simulink model "DRI_furnace"  (R2023b)
settings: Solver=ode15s  StartTime=0.0  StopTime=3600*24
values from neighbouring files (symbols this model uses):
  a_b = 6*(1-eps_bed)/(r_p*2)    (= 200)    [DRI_furnace_loader.m]
  A_furnace = pi*r_furnace^2    (= 23.7582944428)    [DRI_furnace_loader.m]
  A_furnace_pel = A_furnace*(1-eps_bed)    (= 11.8791472214)    [DRI_furnace_loader.m]
  A_wall = (2*pi*r_furnace*dz)    [DRI_furnace_loader.m]
  c_CH4init = interp1([1:1:length(c_CH4init)],c_CH4init, linspace(1,length(c_CH4init),n_furnace))    [DRI_furnace_loader.m]    (also in inital_conditions.m = out.CH4_conc.data(end,:); initcond.mat = [1.85705986545 1.89555733619 1.89749367615 1.89250716351 1.8; initcond_H2.mat = [-5.10200321778e-23 -5.14631233267e-23 -5.19105613109e-23 -5; initcond_NG.mat = [1.53547326032 1.50495486962 1.48970115024 1.4755028102 1.46)
  c_Cinit = interp1([1:1:length(c_Cinit)],c_Cinit, linspace(1,length(c_Cinit),n_furnace))    [DRI_furnace_loader.m]    (also in inital_conditions.m = out.C_conc.data(end,:); initcond.mat = [3.21457388191e-26 -1.33944556404e-26 -9.41053781484e-33 -9.; initcond_H2.mat = [-3.07981965757e-283 -7.05821276017e-284 -1.12151880238e-284; initcond_NG.mat = [40.5707549093 38.5039319297 36.8451113121 35.2570306703 33.)
  c_CO2init = interp1([1:1:length(c_CO2init)],c_CO2init, linspace(1,length(c_CO2init),n_furnace))    [DRI_furnace_loader.m]    (also in inital_conditions.m = out.CO2_conc.data(end,:); initcond.mat = [0.424855142623 0.487573768012 0.610878568601 0.778581871411; initcond_H2.mat = [8.08256932825e-22 8.11925418298e-22 8.15917924386e-22 8.201; initcond_NG.mat = [0.33936960913 0.362161667495 0.389241162314 0.417886502664 )
  c_COinit = interp1([1:1:length(c_COinit)],c_COinit, linspace(1,length(c_COinit),n_furnace))    [DRI_furnace_loader.m]    (also in inital_conditions.m = out.CO_conc.data(end,:); initcond.mat = [5.62429774676 5.68698007947 5.56998267729 5.3860363993 5.16; initcond_H2.mat = [-3.5707332813e-22 -3.59888147715e-22 -3.62743836785e-22 -3.; initcond_NG.mat = [7.01547259829 7.0384402498 7.00998897858 6.97797046171 6.94)
  c_Fe2O3init = interp1([1:1:length(c_Fe2O3init)],c_Fe2O3init, linspace(1,length(c_Fe2O3init),n_furnace))    [DRI_furnace_loader.m]    (also in inital_conditions.m = out.Fe2O3_conc.data(end,:); initcond.mat = [845.154140842 845.181508816 845.220501809 845.323312901 845; initcond_H2.mat = [-0.0380770099519 -0.0370367139242 -0.0360185883395 -0.03502; initcond_NG.mat = [-0.0405281021674 -0.0396025120519 -0.0386898228266 -0.03778)
  c_Fe3O4init = interp1([1:1:length(c_Fe3O4init)],c_Fe3O4init, linspace(1,length(c_Fe3O4init),n_furnace))    [DRI_furnace_loader.m]    (also in inital_conditions.m = out.Fe3O4_conc.data(end,:); initcond.mat = [826.123395955 826.094631755 826.211564736 834.377927258 899; initcond_H2.mat = [0.0321426182211 0.0314818734285 0.030826675132 0.0301767421; initcond_NG.mat = [0.0360465051239 0.0353534026747 0.0346647730928 0.033980211)
  c_Feinit = interp1([1:1:length(c_Feinit)],c_Feinit, linspace(1,length(c_Feinit),n_furnace))    [DRI_furnace_loader.m]    (also in inital_conditions.m = out.Fe_conc.data(end,:); initcond.mat = [836.997845525 830.524010614 758.675200979 644.11637995 545.; initcond_H2.mat = [2198.89990701 2151.53921086 2100.32127816 2045.76128409 198; initcond_NG.mat = [2217.04023267 2190.22219582 2162.02573698 2132.25158626 210)
  c_FeOinit = interp1([1:1:length(c_FeOinit)],c_FeOinit, linspace(1,length(c_FeOinit),n_furnace))    [DRI_furnace_loader.m]    (also in inital_conditions.m = out.FeO_conc.data(end,:); initcond.mat = [523.921847425 532.250412357 624.547839148 764.836368397 835; initcond_H2.mat = [239.269098944 300.197811145 366.088832018 436.279393422 510; initcond_NG.mat = [215.930334993 250.431267245 286.705532207 325.009485154 365)
  c_H2init = interp1([1:1:length(c_H2init)],c_H2init, linspace(1,length(c_H2init),n_furnace))    [DRI_furnace_loader.m]    (also in inital_conditions.m = out.H2_conc.data(end,:); initcond.mat = [8.579601171 8.64686368664 8.51185743267 8.39999947053 8.265; initcond_H2.mat = [17.2543528358 17.2782610911 17.296864644 17.3099892036 17.3; initcond_NG.mat = [11.1435961113 11.2383917061 11.232749456 11.2204098296 11.2)
  c_H2Oinit = interp1([1:1:length(c_H2Oinit)],c_H2Oinit, linspace(1,length(c_H2Oinit),n_furnace))    [DRI_furnace_loader.m]    (also in inital_conditions.m = out.H2O_conc.data(end,:); initcond.mat = [0.757633216435 0.883934685646 1.02867679163 1.11546273638 1; initcond_H2.mat = [0.442325343528 0.548013106661 0.662035872616 0.783558475201; initcond_NG.mat = [0.493575761349 0.511052154474 0.544598386657 0.580268512829)
  c_N2init = interp1([1:1:length(c_N2init)],c_N2init, linspace(1,length(c_N2init),n_furnace))    [DRI_furnace_loader.m]    (also in inital_conditions.m = out.N2_conc.data(end,:); initcond.mat = [0.304985476887 0.311307927602 0.311625933271 0.310806996864; initcond_H2.mat = [0.335892697728 0.338352501527 0.340869822099 0.343425499389; initcond_NG.mat = [0.34370092648 0.344898196415 0.344837358554 0.344718971495 )
  DRIflow = 45.1    [DRI_furnace_loader.m]
  dz = flip(diff(dzfun))    [DRI_furnace_loader.m]
  eps_bed = 0.5    [DRI_furnace_loader.m]
  MM_C = 12.011/1000    (= 0.012011)    [DRI_furnace_loader.m]
  MM_CH4 = 16.04    [DRI_furnace_loader.m]
  MM_CO = 28.01    [DRI_furnace_loader.m]
  MM_CO2 = 44.01    [DRI_furnace_loader.m]
  MM_Fe = 55.845/1000    (= 0.055845)    [DRI_furnace_loader.m]    (also in iron_props.m)
  MM_Fe2O3 = 159.69/1000    (= 0.15969)    [DRI_furnace_loader.m]    (also in iron_props.m)
  MM_Fe3O4 = 251.53/1000    (= 0.25153)    [DRI_furnace_loader.m]    (also in iron_props.m)
  MM_FeO = 71.844/1000    (= 0.071844)    [DRI_furnace_loader.m]    (also in iron_props.m)
  MM_Gan = 60.08/1000    (= 0.06008)    [DRI_furnace_loader.m]
  MM_H2 = 2.016    [DRI_furnace_loader.m]
  MM_H2O = 18.015    [DRI_furnace_loader.m]
  MM_N2 = 28.013    [DRI_furnace_loader.m]
  mol_Fe2O3init = rho_p*0.9665/MM_Fe2O3*V_s(2:end)    [DRI_furnace_loader.m]    (also in inital_conditions.m = out.mol_Fe2O3init.data(end,:); initcond.mat = [61783.2992712 61783.2992712 61783.2992712 61783.2992712 617)
  n_furnace = 25    [DRI_furnace_loader.m]
  ndotinit = interp1([1:1:length(ndotinit)],ndotinit, linspace(1,length(ndotinit),n_furnace))    [DRI_furnace_loader.m]    (also in inital_conditions.m = out.ndot.data(end,:); initcond.mat = [2210.71780913 2256.54672706 2258.85182304 2252.91568039 224; initcond_H2.mat = [2085.86199266 2093.15115329 2100.66626347 2108.33970255 211; initcond_NG.mat = [2330.74775425 2364.28126123 2378.87094646 2385.81987377 238)
  nr1init = ones(size(T_ginit))*33375    [DRI_furnace_loader.m]    (also in inital_conditions.m = out.nr1.data(end,:); initcond.mat = [61803.8716376 61802.685448 61800.9961847 61796.5422507 6178; initcond_H2.mat = [17138.8276975 17138.822469 17138.817352 17138.8123408 17138; initcond_NG.mat = [34277.6800528 34277.6707483 34277.6615734 34277.652487 3427)
  nr2init = ones(size(T_ginit))*22119    [DRI_furnace_loader.m]    (also in inital_conditions.m = out.nr2.data(end,:); initcond.mat = [41188.8753355 41188.8526513 41178.4232644 40740.5447947 379; initcond_H2.mat = [11425.7737029 11425.772508 11425.7713681 11425.7702806 1142; initcond_NG.mat = [22851.536777 22851.5353796 22851.5340375 22851.5327263 2285)
  nr3init = ones(size(T_ginit))*63083    [DRI_furnace_loader.m]    (also in inital_conditions.m = out.nr3.data(end,:); initcond.mat = [123566.152328 121180.275703 99887.5755955 72587.2577367 536; initcond_H2.mat = [31604.1937028 30923.4912249 30187.3497294 29403.1736897 285; initcond_NG.mat = [63729.8393954 62958.9426131 62148.4224578 61292.5508252 603)
  R = 8.314    [Bou.m]    (also in DRI_furnace_loader.m; G_CO.m; MD.m; SMR.m)
  r_furnace = 2.75    [DRI_furnace_loader.m]
  r_p = 15e-3/2    (= 0.0075)    [DRI_furnace_loader.m]
  Reducerflow = 2228.1*(x_H2in*MM_H2 + x_COin*MM_CO + x_H2Oin*MM_H2O +x_CO2in*MM_CO2 + x_N2in*MM_N2 + x_CH4in*MM_CH4)/1000    (= 31.1426394672)    [DRI_furnace_loader.m]
  rho_p = 3528    [DRI_furnace_loader.m]
  T_ginit = interp1([1:1:length(T_ginit)],T_ginit, linspace(1,length(T_ginit),n_furnace))    [DRI_furnace_loader.m]    (also in inital_conditions.m = out.T_g.data(end,:); initcond.mat = [1196.67659973 1106.80014704 1071.61124107 1050.32194229 103; initcond_H2.mat = [1206.04002008 1196.92003246 1187.72467669 1178.52571193 116; initcond_NG.mat = [1059.94701026 1050.97990802 1047.95611626 1045.20600654 104)
  T_sinit = interp1([1:1:length(T_sinit)],T_sinit, linspace(1,length(T_sinit),n_furnace))    [DRI_furnace_loader.m]    (also in inital_conditions.m = out.T_s.data(end,:); initcond.mat = [1154.91557113 1100.93660653 1069.19977285 1049.37027984 104; initcond_H2.mat = [1198.21532505 1188.90892541 1179.58573027 1170.31082456 116; initcond_NG.mat = [1055.14966191 1048.70059171 1045.82868823 1043.13322913 104)
  V_g = (4/3)*pi*r_p^3*n_pellets_dz*(eps_bed/(1-eps_bed))    [DRI_furnace_loader.m]
  V_p = 4/3*pi*r_p^3    (= 1.76714586764e-06)    [DRI_furnace_loader.m]
  V_s = (4/3)*pi*r_p^3*n_pellets_dz    [DRI_furnace_loader.m]
  x_CH4in = 0.105824828    [DRI_furnace_loader.m]
  x_CO2in = 0.024    [DRI_furnace_loader.m]
  x_COin = 0.320711862    [DRI_furnace_loader.m]
  x_H2in = 0.489526511    [DRI_furnace_loader.m]
  x_H2Oin = 0.042557156    [DRI_furnace_loader.m]
  x_N2in = 0.017379642    [DRI_furnace_loader.m]
libraries: simulink x1
(part 1 of 2)
settings Model: Creator=jimmonen  LastModifiedBy=jimmonen
settings SolverCC: AlgebraicLoopSolver=TrustRegion
settings DebuggingCC: UnconnectedInputMsg=warning  UnconnectedOutputMsg=warning  UnconnectedLineMsg=warning
settings ModelReferenceCC: EnableRefExpFcnMdlSchedulingChecks=on
settings RTWCC: DLArmComputeVersion=19.05

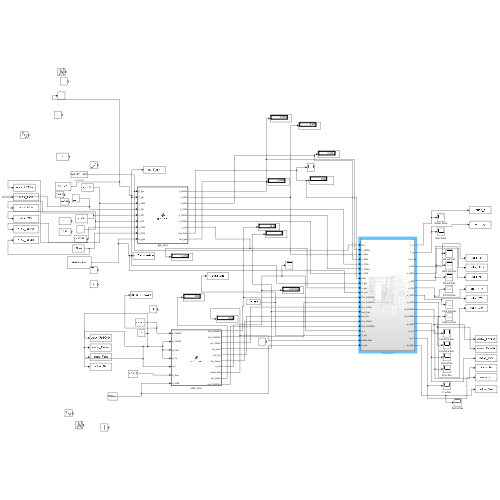
[thumbnail: Simulink's stored preview of the top-level diagram]
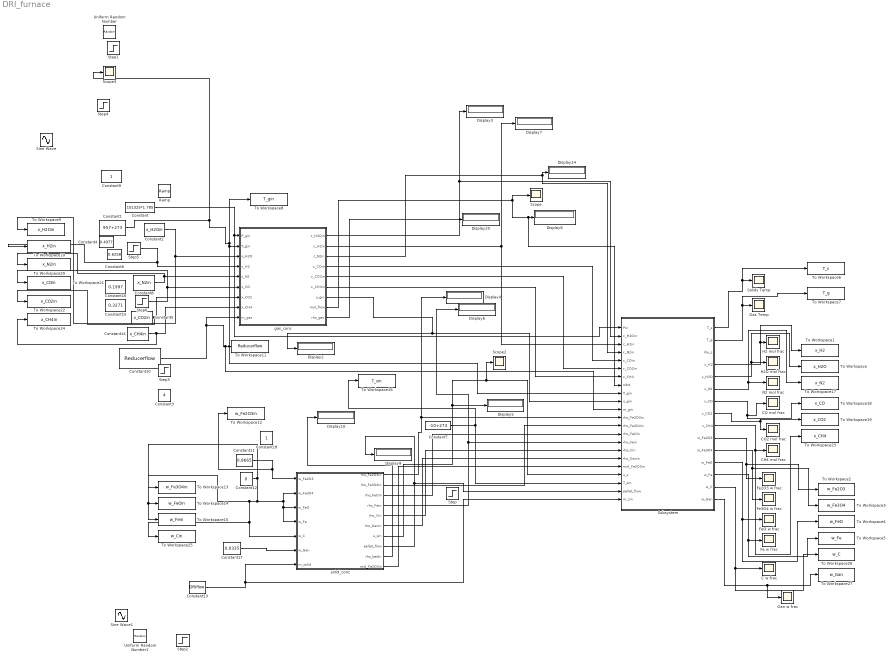
== system DRI_furnace ==
  C w frac : Scope
  CH4 mol frac : Scope
  CO mol frac : Scope
  CO2 mol frac : Scope
  Constant : Constant  Value=101325*1.785
  Constant1 : Constant  Value=957+273
  Constant10 : Constant  Value=Reducerflow
  Constant11 : Constant  Value=0.9665
  Constant12 : Constant  Value=0
  Constant13 : Constant  Value=DRIflow
  Constant14 : Constant  Value=x_CH4in
  Constant15 : Constant  Value=0.3271
  Constant16 : Constant  Value=0.1997
  Constant17 : Constant  Value=0.0335
  Constant18 : Constant
  Constant2 : Constant  Value=x_H2Oin
  Constant3 : Constant  Value=4
  Constant4 : Constant  Value=0.4977
  Constant5 : Constant  Value=x_CO2in
  Constant6 : Constant  Value=0.6258
  Constant7 : Constant  Value=-10+273
  Constant8 : Constant  Value=x_N2in
  Constant9 : Constant
  Display{2..10,14,20} (11 alike) : Display
  Fe w frac : Scope
  Fe2O3 w frac : Scope
  Fe3O4 w frac : Scope
  FeO w frac : Scope
  Gan w frac : Scope
  Gas Temp : Scope
  H2 mol frac : Scope
  H2O mol frac : Scope
  N2 mol frac : Scope
  Ramp : simulink/Sources/Ramp  slope=-5/(3600)  start=3600  InitialOutput=800+273
  Scope : Scope
  Scope2 : Scope
  Scope3 : Scope
  Sine Wave : Sin  Amplitude=2  Bias=Reducerflow  Frequency=1/(3600*0.5)  SampleTime=0
  Sine Wave1 : Sin  Amplitude=15  Bias=52  Frequency=1/(3600*0.5)  SampleTime=0
  Solids Temp : Scope
  Step : Step  Time=3600*6  Before=4750  After=5000  SampleTime=0
  Step1 : Step  Time=3600*1  Before=800+273  After=700+273  SampleTime=0
  Step2 : Step  Time=3600*1  Before=DRIflow  After=DRIflow+25  SampleTime=0
  Step3 : Step  Time=3600*1  Before=Reducerflow  After=14.2236  SampleTime=0
  Step4 : Step  Time=3600*1  Before=0.98  After=0.9  SampleTime=0
  Step5 : Step  Time=3600*1  Before=x_H2in  After=x_H2in  SampleTime=0
  Step6 : Step  Time=3600*1  Before=x_COin  After=x_COin  SampleTime=0
  Subsystem : Subsystem
  To Workspace : ToWorkspace  VariableName=x_H2O  SaveFormat=Timeseries  SampleTime=-1
  To Workspace1 : ToWorkspace  VariableName=x_H2  SaveFormat=Timeseries  SampleTime=-1
  To Workspace10 : ToWorkspace  VariableName=x_H2in  SaveFormat=Timeseries  SampleTime=-1
  To Workspace11 : ToWorkspace  VariableName=Reducerflow  SaveFormat=Timeseries  SampleTime=-1
  To Workspace12 : ToWorkspace  VariableName=w_Fe2O3in  SaveFormat=Timeseries  SampleTime=-1
  To Workspace13 : ToWorkspace  VariableName=w_Fe3O4in  SaveFormat=Timeseries  SampleTime=-1
  To Workspace14 : ToWorkspace  VariableName=w_FeOin  SaveFormat=Timeseries  SampleTime=-1
  To Workspace15 : ToWorkspace  VariableName=w_Fein  SaveFormat=Timeseries  SampleTime=-1
  To Workspace16 : ToWorkspace  VariableName=T_sin  SaveFormat=Timeseries  SampleTime=-1
  To Workspace17 : ToWorkspace  VariableName=x_N2  SaveFormat=Timeseries  SampleTime=-1
  To Workspace18 : ToWorkspace  VariableName=x_CO  SaveFormat=Timeseries  SampleTime=-1
  To Workspace19 : ToWorkspace  VariableName=x_CO2  SaveFormat=Timeseries  SampleTime=-1
  To Workspace2 : ToWorkspace  VariableName=w_Fe2O3  SaveFormat=Timeseries  SampleTime=-1
  To Workspace20 : ToWorkspace  VariableName=x_N2in  SaveFormat=Timeseries  SampleTime=-1
  To Workspace21 : ToWorkspace  VariableName=x_COin  SaveFormat=Timeseries  SampleTime=-1
  To Workspace22 : ToWorkspace  VariableName=x_CO2in  SaveFormat=Timeseries  SampleTime=-1
  To Workspace23 : ToWorkspace  VariableName=x_CH4  SaveFormat=Timeseries  SampleTime=-1
  To Workspace24 : ToWorkspace  VariableName=x_CH4in  SaveFormat=Timeseries  SampleTime=-1
  To Workspace25 : ToWorkspace  VariableName=w_Cin  SaveFormat=Timeseries  SampleTime=-1
  To Workspace26 : ToWorkspace  VariableName=w_C  SaveFormat=Timeseries  SampleTime=-1
  To Workspace27 : ToWorkspace  VariableName=w_Gan  SaveFormat=Timeseries  SampleTime=-1
  To Workspace3 : ToWorkspace  VariableName=w_Fe3O4  SaveFormat=Timeseries  SampleTime=-1
  To Workspace4 : ToWorkspace  VariableName=w_FeO  SaveFormat=Timeseries  SampleTime=-1
  To Workspace5 : ToWorkspace  VariableName=w_Fe  SaveFormat=Timeseries  SampleTime=-1
  To Workspace6 : ToWorkspace  VariableName=T_s  SaveFormat=Timeseries  SampleTime=-1
  To Workspace7 : ToWorkspace  VariableName=T_g  SaveFormat=Timeseries  SampleTime=-1
  To Workspace8 : ToWorkspace  VariableName=T_gin  SaveFormat=Timeseries  SampleTime=-1
  To Workspace9 : ToWorkspace  VariableName=x_H2Oin  SaveFormat=Timeseries  SampleTime=-1
  Uniform Random Number : UniformRandomNumber  Minimum=800  Maximum=1000  SampleTime=3600
  Uniform Random Number1 : UniformRandomNumber  Minimum=DRIflow -7  Maximum=DRIflow +7  SampleTime=3600
  gas_conc : MATLAB Function  TreatAsAtomicUnit=on
  solid_conc : MATLAB Function  TreatAsAtomicUnit=on
  wires:
  gas_conc/1(c_H2Oin) -> Display3/1, Subsystem/2(c_H2Oin)
  gas_conc/2(c_H2in) -> Display7/1, Subsystem/3(c_H2in)
  gas_conc/3(c_N2in) -> Display14/1, Subsystem/4(c_N2in)
  solid_conc/1(rho_Fe2O3in) -> Display4/1, Subsystem/12(rho_Fe2O3in)
  Constant1/1 -> Subsystem/9(T_gin), gas_conc/2(T_gin), To Workspace8/1, Scope3/1
  Constant/1 -> Subsystem/1(Pin), gas_conc/1(P_gin)
  Constant10/1 -> gas_conc/9(m_gas), To Workspace11/1, Subsystem/11(m_gin)
  gas_conc/7(u_gin) -> Subsystem/10(u_gin), Display2/1
  Constant11/1 -> solid_conc/1(w_Fe2O3), To Workspace12/1
  solid_conc/4(rho_Fein) -> Display6/1, Subsystem/15(rho_Fein)
  solid_conc/7(u_sin) -> Scope2/1, Subsystem/19(u_s), Display5/1
  solid_conc/8(pellet_flow) -> Display9/1, Subsystem/21(pellet_flow)
  gas_conc/8(mol_flow) -> Display8/1, Subsystem/8(ndot), Scope/1
  solid_conc/9(rho_bedin) -> Display10/1
  gas_conc/9(rho_gas) -> Display20/1
  Subsystem/2(T_g) -> To Workspace7/1, Gas Temp/1
  Subsystem/1(T_s) -> To Workspace6/1, Solids Temp/1
  Constant7/1 -> To Workspace16/1, Subsystem/20(T_sin)
  solid_conc/2(rho_Fe3O4in) -> Subsystem/13(rho_Fe3O4in)
  solid_conc/3(rho_FeOin) -> Subsystem/14(rho_FeOin)
  Constant13/1 -> solid_conc/7(m_solid), Subsystem/22(m_sin)
  gas_conc/4(c_COin) -> Subsystem/5(c_COin)
  gas_conc/5(c_CO2in) -> Subsystem/6(c_CO2in)
  Step6/1 -> To Workspace21/1, gas_conc/6(x_CO)
  Constant5/1 -> gas_conc/7(x_CO2), To Workspace22/1
  Constant8/1 -> To Workspace20/1, gas_conc/5(x_N2)
  Step5/1 -> To Workspace10/1, gas_conc/4(x_H2)
  Constant2/1 -> To Workspace9/1, gas_conc/3(x_H2O)
  Subsystem/4(x_H2) -> To Workspace1/1, H2 mol frac/1
  Subsystem/5(x_H2O) -> To Workspace/1, H2O mol frac/1
  Subsystem/6(x_N2) -> To Workspace17/1, N2 mol frac/1
  Subsystem/7(x_CO) -> To Workspace18/1, CO mol frac/1
  Subsystem/8(x_CO2) -> CO2 mol frac/1, To Workspace19/1
  Subsystem/10(w_Fe2O3) -> Fe2O3 w frac/1, To Workspace2/1
  Subsystem/11(w_Fe3O4) -> Fe3O4 w frac/1, To Workspace3/1
  Subsystem/13(w_Fe) -> To Workspace5/1, Fe w frac/1
  Subsystem/12(w_FeO) -> To Workspace4/1, FeO w frac/1
  Subsystem/9(x_CH4) -> To Workspace23/1, CH4 mol frac/1
  Constant14/1 -> To Workspace24/1, gas_conc/8(x_CH4)
  gas_conc/6(c_CH4in) -> Subsystem/7(c_CH4)
  solid_conc/5(rho_Cin) -> Subsystem/16(rho_Cin)
  solid_conc/6(rho_Ganin) -> Subsystem/17(rho_Ganin)
  Constant12/1 -> solid_conc/5(w_C), To Workspace25/1, To Workspace15/1, To Workspace14/1, solid_conc/4(w_Fe), solid_conc/3(w_FeO), solid_conc/2(w_Fe3O4), To Workspace13/1
  Subsystem/14(w_C) -> To Workspace26/1, C w frac/1
  Constant17/1 -> solid_conc/6(w_Gan)
  Subsystem/15(w_Gan) -> Gan w frac/1, To Workspace27/1
  solid_conc/10(mol_Fe2O3in) -> Subsystem/18(mol_Fe2O3in)

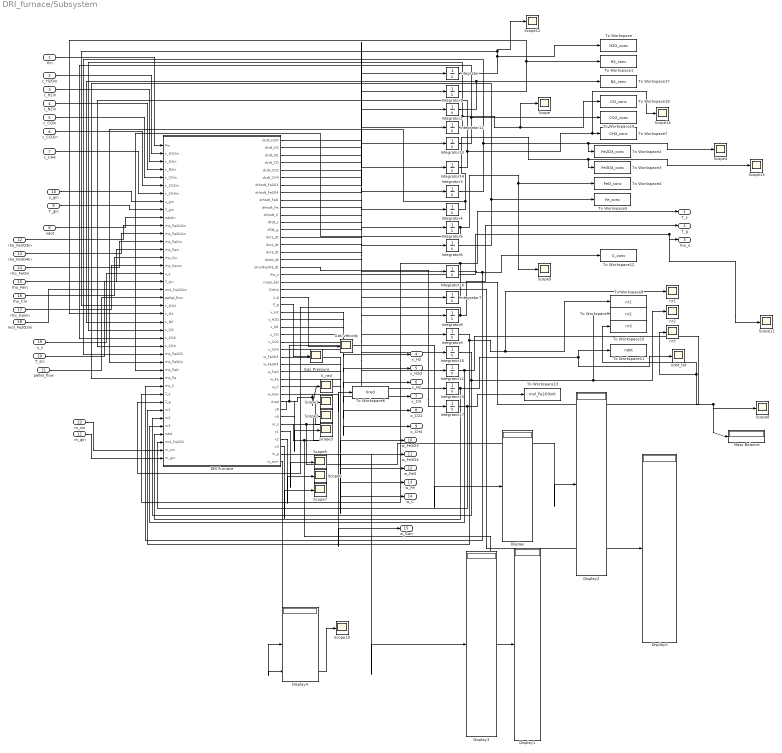
== system DRI_furnace/Subsystem ==
  Pin : Inport
  c_H2Oin : Inport  Port=2
  c_H2in : Inport  Port=3
  c_N2in : Inport  Port=4
  c_COin : Inport  Port=5
  c_CO2in : Inport  Port=6
  c_CH4 : Inport  Port=7
  ndot : Inport  Port=8
  T_gin : Inport  Port=9
  u_gin : Inport  Port=10
  m_gin : Inport  Port=11
  rho_Fe2O3in : Inport  Port=12
  rho_Fe3O4in : Inport  Port=13
  rho_FeOin : Inport  Port=14
  rho_Fein : Inport  Port=15
  rho_Cin : Inport  Port=16
  rho_Ganin : Inport  Port=17
  mol_Fe2O3in : Inport  Port=18
  u_s : Inport  Port=19
  T_sin : Inport  Port=20
  pellet_flow : Inport  Port=21
  m_sin : Inport  Port=22
  DRI Furnace : MATLAB Function  TreatAsAtomicUnit=on
  Display{,1..5} (6 alike) : Display
  Gas Pressure : Scope
  Gas Velocity : Scope
  Integrator : Integrator  InitialCondition=c_H2Oinit
  Integrator1 : Integrator  InitialCondition=c_H2init
  Integrator10 : Integrator  InitialCondition=nr2init
  Integrator11 : Integrator  InitialCondition=nr3init
  Integrator12 : Integrator  InitialCondition=c_COinit
  Integrator13 : Integrator  InitialCondition=c_CO2init
  Integrator14 : Integrator  InitialCondition=c_CH4init
  Integrator15 : Integrator  InitialCondition=ndotinit
  Integrator16 : Integrator  InitialCondition=c_Cinit
  Integrator17 : Integrator  InitialCondition=mol_Fe2O3init
  Integrator2 : Integrator  InitialCondition=c_N2init
  Integrator3 : Integrator  InitialCondition=c_Fe2O3init
  Integrator4 : Integrator  InitialCondition=c_Fe3O4init
  Integrator5 : Integrator  InitialCondition=c_FeOinit
  Integrator6 : Integrator  InitialCondition=c_Feinit
  Integrator7 : Integrator  InitialCondition=T_sinit
  Integrator8 : Integrator  InitialCondition=T_ginit
  Integrator9 : Integrator  InitialCondition=nr1init
  Mass Balance : Display
  Scope{,1..14} (15 alike) : Scope
  To Workspace : ToWorkspace  VariableName=H2O_conc  SaveFormat=Timeseries  SampleTime=-1
  To Workspace1 : ToWorkspace  VariableName=H2_conc  SaveFormat=Timeseries  SampleTime=-1
  To Workspace10 : ToWorkspace  VariableName=nr3  SaveFormat=Timeseries  SampleTime=-1
  To Workspace11 : ToWorkspace  VariableName=ndot  SaveFormat=Timeseries  SampleTime=-1
  To Workspace12 : ToWorkspace  VariableName=C_conc  SaveFormat=Timeseries  SampleTime=-1
  To Workspace13 : ToWorkspace  VariableName=mol_Fe2O3init  SaveFormat=Timeseries  SampleTime=-1
  To Workspace17 : ToWorkspace  VariableName=N2_conc  SaveFormat=Timeseries  SampleTime=-1
  To Workspace18 : ToWorkspace  VariableName=CO_conc  SaveFormat=Timeseries  SampleTime=-1
  To Workspace19 : ToWorkspace  VariableName=CO2_conc  SaveFormat=Timeseries  SampleTime=-1
  To Workspace2 : ToWorkspace  VariableName=Fe2O3_conc  SaveFormat=Timeseries  SampleTime=-1
  To Workspace3 : ToWorkspace  VariableName=Fe3O4_conc  SaveFormat=Timeseries  SampleTime=-1
  To Workspace4 : ToWorkspace  VariableName=FeO_conc  SaveFormat=Timeseries  SampleTime=-1
  To Workspace5 : ToWorkspace  VariableName=Fe_conc  SaveFormat=Timeseries  SampleTime=-1
  To Workspace6 : ToWorkspace  VariableName=Xred  SaveFormat=Timeseries  SampleTime=-1
  To Workspace7 : ToWorkspace  VariableName=CH4_conc  SaveFormat=Timeseries  SampleTime=-1
  To Workspace8 : ToWorkspace  VariableName=nr1  SaveFormat=Timeseries  SampleTime=-1
  To Workspace9 : ToWorkspace  VariableName=nr2  SaveFormat=Timeseries  SampleTime=-1
  X_red : Scope
  ndot_tot : Scope
  nr1 : Scope
  nr2 : Scope
  nr3 : Scope
  T_s : Outport
  T_g : Outport  Port=2
  rho_s : Outport  Port=3
  x_H2 : Outport  Port=4
  x_H2O : Outport  Port=5
  x_N2 : Outport  Port=6
  x_CO : Outport  Port=7
  x_CO2 : Outport  Port=8
  x_CH4 : Outport  Port=9
  w_Fe2O3 : Outport  Port=10
  w_Fe3O4 : Outport  Port=11
  w_FeO : Outport  Port=12
  w_Fe : Outport  Port=13
  w_C : Outport  Port=14
  w_Gan : Outport  Port=15
  wires:
  Integrator8/1 -> T_g/1, DRI Furnace/33(T_g)
  DRI Furnace/2(dcdt_H2) -> Integrator1/1
  Integrator10/1 -> To Workspace9/1, nr2/1, DRI Furnace/35(nr2)
  Integrator1/1 -> To Workspace1/1, DRI Furnace/22(c_H2)
  m_sin/1 -> DRI Furnace/39(m_sin)
  pellet_flow/1 -> DRI Furnace/20(pellet_flow)
  DRI Furnace/3(dcdt_N2) -> Integrator2/1
  Integrator9/1 -> To Workspace8/1, nr1/1, DRI Furnace/34(nr1)
  DRI Furnace/9(drhodt_FeO) -> Integrator5/1
  DRI Furnace/1(dcdt_H2O) -> Integrator/1
  rho_Fe2O3in/1 -> DRI Furnace/11(rho_Fe2O3in)
  DRI Furnace/10(drhodt_Fe) -> Integrator6/1
  Integrator7/1 -> T_s/1, DRI Furnace/32(T_s)
  Integrator4/1 -> Scope13/1, To Workspace3/1, DRI Furnace/28(rho_Fe3O4)
  DRI Furnace/7(drhodt_Fe2O3) -> Integrator3/1
  Integrator3/1 -> DRI Furnace/27(rho_Fe2O3), Scope4/1, To Workspace2/1
  DRI Furnace/13(dTdt_g) -> Integrator8/1
  DRI Furnace/15(dnr2_dt) -> Integrator10/1
  Integrator11/1 -> To Workspace10/1, nr3/1, DRI Furnace/36(nr3)
  DRI Furnace/16(dnr3_dt) -> Integrator11/1
  ndot/1 -> DRI Furnace/10(ndotin)
  T_sin/1 -> DRI Furnace/18(T_sin)
  DRI Furnace/12(dTdt_s) -> Integrator7/1
  Integrator6/1 -> To Workspace5/1, DRI Furnace/30(rho_Fe)
  rho_Fe3O4in/1 -> DRI Furnace/12(rho_Fe3O4in)
  DRI Furnace/20(mass_bal) -> Mass Balance/1, Scope8/1
  T_gin/1 -> DRI Furnace/9(T_gin)
  Integrator2/1 -> To Workspace17/1, DRI Furnace/23(c_N2)
  DRI Furnace/14(dnr1_dt) -> Integrator9/1
  rho_Fein/1 -> DRI Furnace/14(rho_Fein)
  Integrator/1 -> Scope12/1, DRI Furnace/21(c_H2O), To Workspace/1
  u_s/1 -> DRI Furnace/17(u_s)
  DRI Furnace/8(drhodt_Fe3O4) -> Integrator4/1
  c_H2Oin/1 -> DRI Furnace/2(c_H2Oin)
  m_gin/1 -> DRI Furnace/40(m_gin)
  c_H2in/1 -> DRI Furnace/3(c_H2in)
  u_gin/1 -> DRI Furnace/8(u_gin)
  rho_FeOin/1 -> DRI Furnace/13(rho_FeOin)
  c_N2in/1 -> DRI Furnace/4(c_N2in)
  DRI Furnace/4(dcdt_CO) -> Integrator12/1
  DRI Furnace/5(dcdt_CO2) -> Integrator13/1
  Integrator13/1 -> DRI Furnace/25(c_CO2), To Workspace19/1
  Integrator12/1 -> DRI Furnace/24(c_CO), Scope/1, To Workspace18/1
  c_COin/1 -> DRI Furnace/5(c_COin)
  c_CO2in/1 -> DRI Furnace/6(c_CO2in)
  DRI Furnace/28(x_CO2) -> x_CO2/1
  DRI Furnace/27(x_CO) -> x_CO/1
  Integrator5/1 -> DRI Furnace/29(rho_FeO), Scope9/1, To Workspace4/1
  DRI Furnace/25(x_H2O) -> x_H2O/1
  DRI Furnace/24(x_H2) -> x_H2/1
  DRI Furnace/22(u_g) -> Gas Velocity/1
  DRI Furnace/26(x_N2) -> x_N2/1
  DRI Furnace/30(w_Fe2O3) -> w_Fe2O3/1
  DRI Furnace/31(w_Fe3O4) -> w_Fe3O4/1
  DRI Furnace/32(w_FeO) -> w_FeO/1
  DRI Furnace/33(w_Fe) -> w_Fe/1
  DRI Furnace/23(P_g) -> Gas Pressure/1
  DRI Furnace/38(v9) -> Display2/1, Scope1/1
  DRI Furnace/39(m_s) -> Scope2/1, Display1/1
  DRI Furnace/37(v8) -> Scope3/1, Display/1
  DRI Furnace/41(x2) -> Scope6/1
  DRI Furnace/42(x3) -> Scope7/1
  DRI Furnace/40(x1) -> Scope5/1
  DRI Furnace/43(m_g) -> Display3/1
  DRI Furnace/44(w_sum) -> Scope10/1, Display4/1
  Pin/1 -> DRI Furnace/1(Pin)
  DRI Furnace/36(Xred) -> X_red/1, To Workspace6/1
  c_CH4/1 -> DRI Furnace/7(c_CH4in)
  DRI Furnace/6(dcdt_CH4) -> Integrator14/1
  Integrator14/1 -> Scope14/1, To Workspace7/1, DRI Furnace/26(c_CH4)
  DRI Furnace/29(x_CH4) -> x_CH4/1
  DRI Furnace/17(dntot_dt) -> Integrator15/1
  Integrator15/1 -> ndot_tot/1, To Workspace11/1, DRI Furnace/37(ndot)
  rho_Cin/1 -> DRI Furnace/15(rho_Cin)
  rho_Ganin/1 -> DRI Furnace/16(rho_Ganin)
  DRI Furnace/11(drhodt_C) -> Integrator16/1
  Integrator16/1 -> To Workspace12/1, DRI Furnace/31(rho_C)
  DRI Furnace/34(w_C) -> w_C/1
  DRI Furnace/19(rho_s) -> Scope11/1, rho_s/1
  DRI Furnace/21(Cratio) -> Display5/1
  DRI Furnace/35(w_Gan) -> w_Gan/1
  DRI Furnace/18(dmolFe2O3_dt) -> Integrator17/1
  Integrator17/1 -> To Workspace13/1, DRI Furnace/38(mol_Fe2O3)
  mol_Fe2O3in/1 -> DRI Furnace/19(mol_Fe2O3in)

== matlab function DRI_furnace/gas_conc ==
  data: P_gin input; c_H2Oin output; T_gin input; x_H2O input; x_H2 input; x_N2 input; x_CO input; x_CO2 input; x_CH4 input; m_gas input; c_H2in output; c_N2in output; c_COin output; c_CO2in output; c_CH4in output; A_furnace parameter; R parameter; u_gin output; MM_H2O parameter; MM_N2 parameter; MM_H2 parameter; mol_flow output; eps_bed parameter; rho_gas output; MM_CO parameter; MM_CO2 parameter; MM_CH4 parameter
function [c_H2Oin, c_H2in, c_N2in, c_COin, c_CO2in, c_CH4in, u_gin, mol_flow, rho_gas] = gas_conc(P_gin, T_gin, x_H2O, x_H2, x_N2, x_CO, x_CO2, x_CH4, m_gas,A_furnace, R, MM_H2O, MM_N2, MM_H2, eps_bed, MM_CO, MM_CO2, MM_CH4)

%toal molar concentration using ideal gas law
ct = P_gin/(R*T_gin); %mol/m^3 total

%molar concentrations of each gas species in
c_H2Oin = ct * x_H2O; %mol/m^3
c_H2in = ct * x_H2; %mol/m^3
c_N2in = ct * x_N2; %mol/m^3
c_COin = ct * x_CO; %mol/m^3
c_CO2in = ct * x_CO2; %mol/m^3
c_CH4in = ct * x_CH4; %mol/m^3


rho_H2Oin = c_H2Oin*MM_H2O/1000; %kg/m^3 total
rho_H2in = c_H2in*MM_H2/1000; %kg/m^3
rho_N2in = c_N2in*MM_N2/1000; %kg/m^3
rho_COin = c_COin*MM_CO/1000; %kg/m^3
rho_CO2in = c_CO2in*MM_CO2/1000; %kg/m^3
rho_CH4in = c_CH4in*MM_CO2/1000; %kg/m^3

w_totin = (c_H2in*MM_H2 + c_H2Oin*MM_H2O + c_N2in*MM_N2 + c_COin*MM_CO + c_CO2in*MM_CO2 + c_CH4in*MM_CH4);

w_H2in = c_H2in*MM_H2/w_totin;
w_H2Oin = c_H2Oin*MM_H2O /w_totin;
w_N2in = c_N2in*MM_N2/w_totin;
w_COin = c_COin*MM_CO/w_totin;
w_CO2in = c_CO2in*MM_CO2/w_totin;
w_CH4in = c_CH4in*MM_CH4/w_totin;



mol_flow = m_gas*(w_H2Oin/(MM_H2O/1000) + w_H2in/(MM_H2/1000) + w_N2in/(MM_N2/1000) + w_COin/(MM_CO/1000) + w_CO2in/(MM_CO2/1000) + w_CH4in/(MM_CH4/1000)) ;
rho_gas = rho_H2Oin + rho_H2in + rho_N2in + rho_COin + rho_CO2in + rho_CH4in ; %kg/m^3 of GAS


u_sup = m_gas/(rho_gas*A_furnace);

u_gin = u_sup/eps_bed;


%u_gin = m_gas/rho_gas/(A_furnace*eps_bed); %m/s of gas (interstitial velocity)

%u_gS = u_gin*;
